simulink model "filtros_sb_r2015b"  (R2015b)
settings: Solver=VariableStepAuto  SolverMode=SingleTasking  StartTime=0.0  StopTime=10.0  RelTol=1e-3
(part 1 of 3)
settings Model: Creator=vini  LastModifiedBy=vini
settings DataIOCC: LimitDataPoints=off
settings DebuggingCC: AllowSymbolicDim=on  SFUnexpectedBacktrackingDiag=error  SFNoUnconditionalDefaultTransitionDiag=error
settings ModelReferenceCC: PropagateSignalLabelsOutOfModel=on
settings SFSimCC: SimUseLocalCustomCode=on
settings RTWCC: RTWUseLocalCustomCode=on
settings GRTTargetCC: TargetLangStandard=C99 (ISO)
settings ConfigComp: CovMetricSettings=dwe  CovHtmlReporting=off  CovSaveCumulativeToWorkspaceVar=off  CovSaveSingleToWorkspaceVar=off  CovModelRefEnable=Off  CovExternalEMLEnable=on

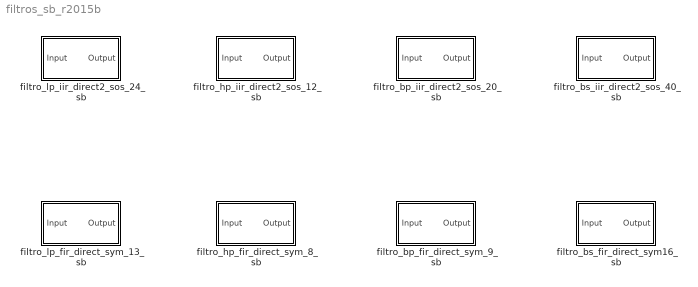
== system filtros_sb_r2015b ==
  filtro_bp_fir_direct_sym_9_sb : Subsystem  Tag=FilterWizardSubSystem
      settings: ErrorFcn=dspFilterRealizedInBasicElemsAlgLoopErrFcnCallback
  filtro_bp_iir_direct2_sos_20_sb : Subsystem  Tag=FilterWizardSubSystem
      settings: ErrorFcn=dspFilterRealizedInBasicElemsAlgLoopErrFcnCallback
  filtro_bs_fir_direct_sym16_sb : Subsystem  Tag=FilterWizardSubSystem
      settings: ErrorFcn=dspFilterRealizedInBasicElemsAlgLoopErrFcnCallback
  filtro_bs_iir_direct2_sos_40_sb : Subsystem  Tag=FilterWizardSubSystem
      settings: ErrorFcn=dspFilterRealizedInBasicElemsAlgLoopErrFcnCallback
  filtro_hp_fir_direct_sym_8_sb : Subsystem  Tag=FilterWizardSubSystem
      settings: ErrorFcn=dspFilterRealizedInBasicElemsAlgLoopErrFcnCallback
  filtro_hp_iir_direct2_sos_12_sb : Subsystem  Tag=FilterWizardSubSystem
      settings: ErrorFcn=dspFilterRealizedInBasicElemsAlgLoopErrFcnCallback
  filtro_lp_fir_direct_sym_13_sb : Subsystem  Tag=FilterWizardSubSystem
      settings: ErrorFcn=dspFilterRealizedInBasicElemsAlgLoopErrFcnCallback
  filtro_lp_iir_direct2_sos_24_sb : Subsystem  Tag=FilterWizardSubSystem
      settings: ErrorFcn=dspFilterRealizedInBasicElemsAlgLoopErrFcnCallback

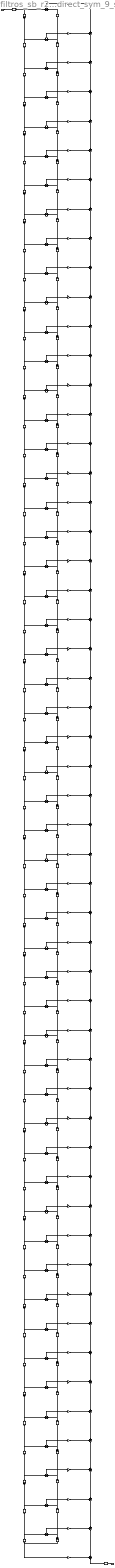
== system filtros_sb_r2015b/filtro_bp_fir_direct_sym_9_sb ==
  Input : Inport
  BodyDelayL{2..53} (52 alike) : Delay  DelayLength=1  InitialCondition=0
  BodyDelayR{2..53} (52 alike) : Delay  DelayLength=1  InitialCondition=0
  BodySumL{2..53} (52 alike) : Sum  Inputs=+|+  AccumDataTypeStr=fixdt(1,17,15)  OutDataTypeStr=fixdt(1,17,15)  RndMeth=Convergent
  BodySumR{2..53} (52 alike) : Sum  Inputs=++|  AccumDataTypeStr=fixdt(1,28,28)  OutDataTypeStr=fixdt(1,28,28)  RndMeth=Convergent
  ConvertIn : DataTypeConversion  OutDataTypeStr=fixdt(1,16,15)  RndMeth=Nearest  SaturateOnIntegerOverflow=on
  ConvertOut : DataTypeConversion  OutDataTypeStr=fixdt(1,28,28)  RndMeth=Convergent
  FootDelayL54 : Delay  DelayLength=1  InitialCondition=0
  FootSumR54 : Sum  Inputs=++|  AccumDataTypeStr=fixdt(1,28,28)  OutDataTypeStr=fixdt(1,28,28)  RndMeth=Convergent
  HeadDelayR1 : Delay  DelayLength=1  InitialCondition=0
  HeadSumL1 : Sum  Inputs=+|+  AccumDataTypeStr=fixdt(1,17,15)  OutDataTypeStr=fixdt(1,17,15)  RndMeth=Convergent
  h(1) : Gain  Gain=0.00100515299929475744  ParamDataTypeStr=fixdt(1,9,13)  OutDataTypeStr=fixdt(1,25,28)  RndMeth=Convergent
  h(10) : Gain  Gain=0.00286815818250266922  ParamDataTypeStr=fixdt(1,9,13)  OutDataTypeStr=fixdt(1,25,28)  RndMeth=Convergent
  h(11) : Gain  Gain=-0.00275820945661910556  ParamDataTypeStr=fixdt(1,9,13)  OutDataTypeStr=fixdt(1,25,28)  RndMeth=Convergent
  h(12) : Gain  Gain=-0.000348548076347779238  ParamDataTypeStr=fixdt(1,9,13)  OutDataTypeStr=fixdt(1,25,28)  RndMeth=Convergent
  h(13) : Gain  Gain=0.00308223640377106858  ParamDataTypeStr=fixdt(1,9,13)  OutDataTypeStr=fixdt(1,25,28)  RndMeth=Convergent
  h(14) : Gain  Gain=-0.00247713159189788274  ParamDataTypeStr=fixdt(1,9,13)  OutDataTypeStr=fixdt(1,25,28)  RndMeth=Convergent
  h(15) : Gain  Gain=-0.000700500797948935394  ParamDataTypeStr=fixdt(1,9,13)  OutDataTypeStr=fixdt(1,25,28)  RndMeth=Convergent
  h(16) : Gain  Gain=0.00291102947938030529  ParamDataTypeStr=fixdt(1,9,13)  OutDataTypeStr=fixdt(1,25,28)  RndMeth=Convergent
  h(17) : Gain  Gain=-0.00190512093037833075  ParamDataTypeStr=fixdt(1,9,13)  OutDataTypeStr=fixdt(1,25,28)  RndMeth=Convergent
  h(18) : Gain  Gain=-0.000876223286937654927  ParamDataTypeStr=fixdt(1,9,13)  OutDataTypeStr=fixdt(1,25,28)  RndMeth=Convergent
  h(19) : Gain  Gain=0.00226433455335455815  ParamDataTypeStr=fixdt(1,9,13)  OutDataTypeStr=fixdt(1,25,28)  RndMeth=Convergent
  h(2) : Gain  Gain=-0.00558254997081729723  ParamDataTypeStr=fixdt(1,9,13)  OutDataTypeStr=fixdt(1,25,28)  RndMeth=Convergent
  h(20) : Gain  Gain=-0.00111255989139955741  ParamDataTypeStr=fixdt(1,9,13)  OutDataTypeStr=fixdt(1,25,28)  RndMeth=Convergent
  h(21) : Gain  Gain=-0.000728999124363284351  ParamDataTypeStr=fixdt(1,9,13)  OutDataTypeStr=fixdt(1,25,28)  RndMeth=Convergent
  h(22) : Gain  Gain=0.00110819121290996431  ParamDataTypeStr=fixdt(1,9,13)  OutDataTypeStr=fixdt(1,25,28)  RndMeth=Convergent
  h(23) : Gain  Gain=-0.000227511078529173545  ParamDataTypeStr=fixdt(1,9,13)  OutDataTypeStr=fixdt(1,25,28)  RndMeth=Convergent
  h(24) : Gain  Gain=-0.000130659589522396947  ParamDataTypeStr=fixdt(1,9,13)  OutDataTypeStr=fixdt(1,25,28)  RndMeth=Convergent
  h(25) : Gain  Gain=-0.000523156580736449479  ParamDataTypeStr=fixdt(1,9,13)  OutDataTypeStr=fixdt(1,25,28)  RndMeth=Convergent
  h(26) : Gain  Gain=0.000595097230863097788  ParamDataTypeStr=fixdt(1,9,13)  OutDataTypeStr=fixdt(1,25,28)  RndMeth=Convergent
  h(27) : Gain  Gain=0.000998204699623622856  ParamDataTypeStr=fixdt(1,9,13)  OutDataTypeStr=fixdt(1,25,28)  RndMeth=Convergent
  h(28) : Gain  Gain=-0.00252037579099768623  ParamDataTypeStr=fixdt(1,9,13)  OutDataTypeStr=fixdt(1,25,28)  RndMeth=Convergent
  h(29) : Gain  Gain=0.00118419786753528396  ParamDataTypeStr=fixdt(1,9,13)  OutDataTypeStr=fixdt(1,25,28)  RndMeth=Convergent
  h(3) : Gain  Gain=-0.000115189176738601603  ParamDataTypeStr=fixdt(1,9,13)  OutDataTypeStr=fixdt(1,25,28)  RndMeth=Convergent
  h(30) : Gain  Gain=0.00267636778181485832  ParamDataTypeStr=fixdt(1,9,13)  OutDataTypeStr=fixdt(1,25,28)  RndMeth=Convergent
  h(31) : Gain  Gain=-0.00472207215493734064  ParamDataTypeStr=fixdt(1,9,13)  OutDataTypeStr=fixdt(1,25,28)  RndMeth=Convergent
  h(32) : Gain  Gain=0.0013923772800106325  ParamDataTypeStr=fixdt(1,9,13)  OutDataTypeStr=fixdt(1,25,28)  RndMeth=Convergent
  h(33) : Gain  Gain=0.00485014717213684207  ParamDataTypeStr=fixdt(1,9,13)  OutDataTypeStr=fixdt(1,25,28)  RndMeth=Convergent
  h(34) : Gain  Gain=-0.0069235701399356555  ParamDataTypeStr=fixdt(1,9,13)  OutDataTypeStr=fixdt(1,25,28)  RndMeth=Convergent
  h(35) : Gain  Gain=0.00111058492648639755  ParamDataTypeStr=fixdt(1,9,13)  OutDataTypeStr=fixdt(1,25,28)  RndMeth=Convergent
  h(36) : Gain  Gain=0.00739537400156014147  ParamDataTypeStr=fixdt(1,9,13)  OutDataTypeStr=fixdt(1,25,28)  RndMeth=Convergent
  h(37) : Gain  Gain=-0.0089146697340637248  ParamDataTypeStr=fixdt(1,9,13)  OutDataTypeStr=fixdt(1,25,28)  RndMeth=Convergent
  h(38) : Gain  Gain=0.000291547634539236929  ParamDataTypeStr=fixdt(1,9,13)  OutDataTypeStr=fixdt(1,25,28)  RndMeth=Convergent
  h(39) : Gain  Gain=0.0101165373593516666  ParamDataTypeStr=fixdt(1,9,13)  OutDataTypeStr=fixdt(1,25,28)  RndMeth=Convergent
  h(4) : Gain  Gain=0.00166912945599871393  ParamDataTypeStr=fixdt(1,9,13)  OutDataTypeStr=fixdt(1,25,28)  RndMeth=Convergent
  h(40) : Gain  Gain=-0.0104857988001575194  ParamDataTypeStr=fixdt(1,9,13)  OutDataTypeStr=fixdt(1,25,28)  RndMeth=Convergent
  h(41) : Gain  Gain=-0.00104127650841544521  ParamDataTypeStr=fixdt(1,9,13)  OutDataTypeStr=fixdt(1,25,28)  RndMeth=Convergent
  h(42) : Gain  Gain=0.0127989855562083161  ParamDataTypeStr=fixdt(1,9,13)  OutDataTypeStr=fixdt(1,25,28)  RndMeth=Convergent
  h(43) : Gain  Gain=-0.0114759563587348446  ParamDataTypeStr=fixdt(1,9,13)  OutDataTypeStr=fixdt(1,25,28)  RndMeth=Convergent
  h(44) : Gain  Gain=-0.00278510221499259731  ParamDataTypeStr=fixdt(1,9,13)  OutDataTypeStr=fixdt(1,25,28)  RndMeth=Convergent
  h(45) : Gain  Gain=0.0152021800163741443  ParamDataTypeStr=fixdt(1,9,13)  OutDataTypeStr=fixdt(1,25,28)  RndMeth=Convergent
  h(46) : Gain  Gain=-0.0117944650547391772  ParamDataTypeStr=fixdt(1,9,13)  OutDataTypeStr=fixdt(1,25,28)  RndMeth=Convergent
  h(47) : Gain  Gain=-0.0047960103156442415  ParamDataTypeStr=fixdt(1,9,13)  OutDataTypeStr=fixdt(1,25,28)  RndMeth=Convergent
  h(48) : Gain  Gain=0.0171010225526483199  ParamDataTypeStr=fixdt(1,9,13)  OutDataTypeStr=fixdt(1,25,28)  RndMeth=Convergent
  h(49) : Gain  Gain=-0.011405080653360546  ParamDataTypeStr=fixdt(1,9,13)  OutDataTypeStr=fixdt(1,25,28)  RndMeth=Convergent
  h(5) : Gain  Gain=-0.00245594406802915636  ParamDataTypeStr=fixdt(1,9,13)  OutDataTypeStr=fixdt(1,25,28)  RndMeth=Convergent
  h(50) : Gain  Gain=-0.0068708962846339202  ParamDataTypeStr=fixdt(1,9,13)  OutDataTypeStr=fixdt(1,25,28)  RndMeth=Convergent
  h(51) : Gain  Gain=0.0183207654282308771  ParamDataTypeStr=fixdt(1,9,13)  OutDataTypeStr=fixdt(1,25,28)  RndMeth=Convergent
  h(52) : Gain  Gain=-0.0103680972660661636  ParamDataTypeStr=fixdt(1,9,13)  OutDataTypeStr=fixdt(1,25,28)  RndMeth=Convergent
  h(53) : Gain  Gain=-0.00879719931139648879  ParamDataTypeStr=fixdt(1,9,13)  OutDataTypeStr=fixdt(1,25,28)  RndMeth=Convergent
  h(54) : Gain  Gain=0.0187398159211636384  ParamDataTypeStr=fixdt(1,9,13)  OutDataTypeStr=fixdt(1,25,28)  RndMeth=Convergent
  h(6) : Gain  Gain=0.000356865544766645523  ParamDataTypeStr=fixdt(1,9,13)  OutDataTypeStr=fixdt(1,25,28)  RndMeth=Convergent
  h(7) : Gain  Gain=0.00239165624029355917  ParamDataTypeStr=fixdt(1,9,13)  OutDataTypeStr=fixdt(1,25,28)  RndMeth=Convergent
  h(8) : Gain  Gain=-0.00273121981286996232  ParamDataTypeStr=fixdt(1,9,13)  OutDataTypeStr=fixdt(1,25,28)  RndMeth=Convergent
  h(9) : Gain  Gain=4.08985834428046829e-05  ParamDataTypeStr=fixdt(1,9,13)  OutDataTypeStr=fixdt(1,25,28)  RndMeth=Convergent
  Output : Outport
  wires:
  Input/1 -> ConvertIn/1
  HeadSumL1/1 -> h(1)/1
  h(1)/1 -> BodySumR2/2
  HeadDelayR1/1 -> HeadSumL1/2
  ConvertIn/1 -> HeadSumL1/1, BodyDelayL2/1
  BodyDelayL2/1 -> BodySumL2/1, BodyDelayL3/1
  BodySumL2/1 -> h(2)/1
  h(2)/1 -> BodySumR2/1
  BodyDelayR2/1 -> BodySumL2/2, HeadDelayR1/1
  BodySumR2/1 -> BodySumR3/2
  BodyDelayL3/1 -> BodySumL3/1, BodyDelayL4/1
  BodySumL3/1 -> h(3)/1
  h(3)/1 -> BodySumR3/1
  BodyDelayR3/1 -> BodySumL3/2, BodyDelayR2/1
  BodySumR3/1 -> BodySumR4/2
  BodyDelayL4/1 -> BodySumL4/1, BodyDelayL5/1
  BodySumL4/1 -> h(4)/1
  h(4)/1 -> BodySumR4/1
  BodyDelayR4/1 -> BodySumL4/2, BodyDelayR3/1
  BodySumR4/1 -> BodySumR5/2
  BodyDelayL5/1 -> BodySumL5/1, BodyDelayL6/1
  BodySumL5/1 -> h(5)/1
  h(5)/1 -> BodySumR5/1
  BodyDelayR5/1 -> BodySumL5/2, BodyDelayR4/1
  BodySumR5/1 -> BodySumR6/2
  BodyDelayL6/1 -> BodySumL6/1, BodyDelayL7/1
  BodySumL6/1 -> h(6)/1
  h(6)/1 -> BodySumR6/1
  BodyDelayR6/1 -> BodySumL6/2, BodyDelayR5/1
  BodySumR6/1 -> BodySumR7/2
  BodyDelayL7/1 -> BodySumL7/1, BodyDelayL8/1
  BodySumL7/1 -> h(7)/1
  h(7)/1 -> BodySumR7/1
  BodyDelayR7/1 -> BodySumL7/2, BodyDelayR6/1
  BodySumR7/1 -> BodySumR8/2
  BodyDelayL8/1 -> BodySumL8/1, BodyDelayL9/1
  BodySumL8/1 -> h(8)/1
  h(8)/1 -> BodySumR8/1
  BodyDelayR8/1 -> BodySumL8/2, BodyDelayR7/1
  BodySumR8/1 -> BodySumR9/2
  BodyDelayL9/1 -> BodySumL9/1, BodyDelayL10/1
  BodySumL9/1 -> h(9)/1
  h(9)/1 -> BodySumR9/1
  BodyDelayR9/1 -> BodySumL9/2, BodyDelayR8/1
  BodySumR9/1 -> BodySumR10/2
  BodyDelayL10/1 -> BodySumL10/1, BodyDelayL11/1
  BodySumL10/1 -> h(10)/1
  h(10)/1 -> BodySumR10/1
  BodyDelayR10/1 -> BodySumL10/2, BodyDelayR9/1
  BodySumR10/1 -> BodySumR11/2
  BodyDelayL11/1 -> BodySumL11/1, BodyDelayL12/1
  BodySumL11/1 -> h(11)/1
  h(11)/1 -> BodySumR11/1
  BodyDelayR11/1 -> BodySumL11/2, BodyDelayR10/1
  BodySumR11/1 -> BodySumR12/2
  BodyDelayL12/1 -> BodySumL12/1, BodyDelayL13/1
  BodySumL12/1 -> h(12)/1
  h(12)/1 -> BodySumR12/1
  BodyDelayR12/1 -> BodySumL12/2, BodyDelayR11/1
  BodySumR12/1 -> BodySumR13/2
  BodyDelayL13/1 -> BodySumL13/1, BodyDelayL14/1
  BodySumL13/1 -> h(13)/1
  h(13)/1 -> BodySumR13/1
  BodyDelayR13/1 -> BodySumL13/2, BodyDelayR12/1
  BodySumR13/1 -> BodySumR14/2
  BodyDelayL14/1 -> BodySumL14/1, BodyDelayL15/1
  BodySumL14/1 -> h(14)/1
  h(14)/1 -> BodySumR14/1
  BodyDelayR14/1 -> BodySumL14/2, BodyDelayR13/1
  BodySumR14/1 -> BodySumR15/2
  BodyDelayL15/1 -> BodySumL15/1, BodyDelayL16/1
  BodySumL15/1 -> h(15)/1
  h(15)/1 -> BodySumR15/1
  BodyDelayR15/1 -> BodySumL15/2, BodyDelayR14/1
  BodySumR15/1 -> BodySumR16/2
  BodyDelayL16/1 -> BodySumL16/1, BodyDelayL17/1
  BodySumL16/1 -> h(16)/1
  h(16)/1 -> BodySumR16/1
  BodyDelayR16/1 -> BodySumL16/2, BodyDelayR15/1
  BodySumR16/1 -> BodySumR17/2
  BodyDelayL17/1 -> BodySumL17/1, BodyDelayL18/1
  BodySumL17/1 -> h(17)/1
  h(17)/1 -> BodySumR17/1
  BodyDelayR17/1 -> BodySumL17/2, BodyDelayR16/1
  BodySumR17/1 -> BodySumR18/2
  BodyDelayL18/1 -> BodySumL18/1, BodyDelayL19/1
  BodySumL18/1 -> h(18)/1
  h(18)/1 -> BodySumR18/1
  BodyDelayR18/1 -> BodySumL18/2, BodyDelayR17/1
  BodySumR18/1 -> BodySumR19/2
  BodyDelayL19/1 -> BodySumL19/1, BodyDelayL20/1
  BodySumL19/1 -> h(19)/1
  h(19)/1 -> BodySumR19/1
  BodyDelayR19/1 -> BodySumL19/2, BodyDelayR18/1
  BodySumR19/1 -> BodySumR20/2
  BodyDelayL20/1 -> BodySumL20/1, BodyDelayL21/1
  BodySumL20/1 -> h(20)/1
  h(20)/1 -> BodySumR20/1
  BodyDelayR20/1 -> BodySumL20/2, BodyDelayR19/1
  BodySumR20/1 -> BodySumR21/2
  BodyDelayL21/1 -> BodySumL21/1, BodyDelayL22/1
  BodySumL21/1 -> h(21)/1
  h(21)/1 -> BodySumR21/1
  BodyDelayR21/1 -> BodySumL21/2, BodyDelayR20/1
  BodySumR21/1 -> BodySumR22/2
  BodyDelayL22/1 -> BodySumL22/1, BodyDelayL23/1
  BodySumL22/1 -> h(22)/1
  h(22)/1 -> BodySumR22/1
  BodyDelayR22/1 -> BodySumL22/2, BodyDelayR21/1
  BodySumR22/1 -> BodySumR23/2
  BodyDelayL23/1 -> BodySumL23/1, BodyDelayL24/1
  BodySumL23/1 -> h(23)/1
  h(23)/1 -> BodySumR23/1
  BodyDelayR23/1 -> BodySumL23/2, BodyDelayR22/1
  BodySumR23/1 -> BodySumR24/2
  BodyDelayL24/1 -> BodySumL24/1, BodyDelayL25/1
  BodySumL24/1 -> h(24)/1
  h(24)/1 -> BodySumR24/1
  BodyDelayR24/1 -> BodySumL24/2, BodyDelayR23/1
  BodySumR24/1 -> BodySumR25/2
  BodyDelayL25/1 -> BodySumL25/1, BodyDelayL26/1
  BodySumL25/1 -> h(25)/1
  h(25)/1 -> BodySumR25/1
  BodyDelayR25/1 -> BodySumL25/2, BodyDelayR24/1
  BodySumR25/1 -> BodySumR26/2
  BodyDelayL26/1 -> BodySumL26/1, BodyDelayL27/1
  BodySumL26/1 -> h(26)/1
  h(26)/1 -> BodySumR26/1
  BodyDelayR26/1 -> BodySumL26/2, BodyDelayR25/1
  BodySumR26/1 -> BodySumR27/2
  BodyDelayL27/1 -> BodySumL27/1, BodyDelayL28/1
  BodySumL27/1 -> h(27)/1
  h(27)/1 -> BodySumR27/1
  BodyDelayR27/1 -> BodySumL27/2, BodyDelayR26/1
  BodySumR27/1 -> BodySumR28/2
  BodyDelayL28/1 -> BodySumL28/1, BodyDelayL29/1
  BodySumL28/1 -> h(28)/1
  h(28)/1 -> BodySumR28/1
  BodyDelayR28/1 -> BodySumL28/2, BodyDelayR27/1
  BodySumR28/1 -> BodySumR29/2
  BodyDelayL29/1 -> BodySumL29/1, BodyDelayL30/1
  BodySumL29/1 -> h(29)/1
  h(29)/1 -> BodySumR29/1
  BodyDelayR29/1 -> BodySumL29/2, BodyDelayR28/1
  BodySumR29/1 -> BodySumR30/2
  BodyDelayL30/1 -> BodySumL30/1, BodyDelayL31/1
  BodySumL30/1 -> h(30)/1
  h(30)/1 -> BodySumR30/1
  BodyDelayR30/1 -> BodySumL30/2, BodyDelayR29/1
  BodySumR30/1 -> BodySumR31/2
  BodyDelayL31/1 -> BodySumL31/1, BodyDelayL32/1
  BodySumL31/1 -> h(31)/1
  h(31)/1 -> BodySumR31/1
  BodyDelayR31/1 -> BodySumL31/2, BodyDelayR30/1
  BodySumR31/1 -> BodySumR32/2
  BodyDelayL32/1 -> BodySumL32/1, BodyDelayL33/1
  BodySumL32/1 -> h(32)/1
  h(32)/1 -> BodySumR32/1
  BodyDelayR32/1 -> BodySumL32/2, BodyDelayR31/1
  BodySumR32/1 -> BodySumR33/2
  BodyDelayL33/1 -> BodySumL33/1, BodyDelayL34/1
  BodySumL33/1 -> h(33)/1
  h(33)/1 -> BodySumR33/1
  BodyDelayR33/1 -> BodySumL33/2, BodyDelayR32/1
  BodySumR33/1 -> BodySumR34/2
  BodyDelayL34/1 -> BodySumL34/1, BodyDelayL35/1
  BodySumL34/1 -> h(34)/1
  h(34)/1 -> BodySumR34/1
  BodyDelayR34/1 -> BodySumL34/2, BodyDelayR33/1
  BodySumR34/1 -> BodySumR35/2
  BodyDelayL35/1 -> BodySumL35/1, BodyDelayL36/1
  BodySumL35/1 -> h(35)/1
  h(35)/1 -> BodySumR35/1
  BodyDelayR35/1 -> BodySumL35/2, BodyDelayR34/1
  BodySumR35/1 -> BodySumR36/2
  BodyDelayL36/1 -> BodySumL36/1, BodyDelayL37/1
  BodySumL36/1 -> h(36)/1
  h(36)/1 -> BodySumR36/1
  BodyDelayR36/1 -> BodySumL36/2, BodyDelayR35/1
  BodySumR36/1 -> BodySumR37/2
  BodyDelayL37/1 -> BodySumL37/1, BodyDelayL38/1
  BodySumL37/1 -> h(37)/1
  h(37)/1 -> BodySumR37/1
  BodyDelayR37/1 -> BodySumL37/2, BodyDelayR36/1
  BodySumR37/1 -> BodySumR38/2
  BodyDelayL38/1 -> BodySumL38/1, BodyDelayL39/1
  BodySumL38/1 -> h(38)/1
  h(38)/1 -> BodySumR38/1
  BodyDelayR38/1 -> BodySumL38/2, BodyDelayR37/1
  BodySumR38/1 -> BodySumR39/2
  BodyDelayL39/1 -> BodySumL39/1, BodyDelayL40/1
  BodySumL39/1 -> h(39)/1
  h(39)/1 -> BodySumR39/1
  BodyDelayR39/1 -> BodySumL39/2, BodyDelayR38/1
  BodySumR39/1 -> BodySumR40/2
  BodyDelayL40/1 -> BodySumL40/1, BodyDelayL41/1
  BodySumL40/1 -> h(40)/1
  h(40)/1 -> BodySumR40/1
  BodyDelayR40/1 -> BodySumL40/2, BodyDelayR39/1
  BodySumR40/1 -> BodySumR41/2
  BodyDelayL41/1 -> BodySumL41/1, BodyDelayL42/1
  BodySumL41/1 -> h(41)/1
  h(41)/1 -> BodySumR41/1
  BodyDelayR41/1 -> BodySumL41/2, BodyDelayR40/1
  BodySumR41/1 -> BodySumR42/2
  BodyDelayL42/1 -> BodySumL42/1, BodyDelayL43/1
  BodySumL42/1 -> h(42)/1
  h(42)/1 -> BodySumR42/1
  BodyDelayR42/1 -> BodySumL42/2, BodyDelayR41/1
  BodySumR42/1 -> BodySumR43/2
  BodyDelayL43/1 -> BodySumL43/1, BodyDelayL44/1
  BodySumL43/1 -> h(43)/1
  h(43)/1 -> BodySumR43/1
  BodyDelayR43/1 -> BodySumL43/2, BodyDelayR42/1
  BodySumR43/1 -> BodySumR44/2
  BodyDelayL44/1 -> BodySumL44/1, BodyDelayL45/1
  BodySumL44/1 -> h(44)/1
  h(44)/1 -> BodySumR44/1
  BodyDelayR44/1 -> BodySumL44/2, BodyDelayR43/1
  BodySumR44/1 -> BodySumR45/2
  BodyDelayL45/1 -> BodySumL45/1, BodyDelayL46/1
  BodySumL45/1 -> h(45)/1
  h(45)/1 -> BodySumR45/1
  BodyDelayR45/1 -> BodySumL45/2, BodyDelayR44/1
  BodySumR45/1 -> BodySumR46/2
  BodyDelayL46/1 -> BodySumL46/1, BodyDelayL47/1
  BodySumL46/1 -> h(46)/1
  h(46)/1 -> BodySumR46/1
  BodyDelayR46/1 -> BodySumL46/2, BodyDelayR45/1
  BodySumR46/1 -> BodySumR47/2
  BodyDelayL47/1 -> BodySumL47/1, BodyDelayL48/1
  BodySumL47/1 -> h(47)/1
  h(47)/1 -> BodySumR47/1
  BodyDelayR47/1 -> BodySumL47/2, BodyDelayR46/1
  BodySumR47/1 -> BodySumR48/2
  BodyDelayL48/1 -> BodySumL48/1, BodyDelayL49/1
  BodySumL48/1 -> h(48)/1
  h(48)/1 -> BodySumR48/1
  BodyDelayR48/1 -> BodySumL48/2, BodyDelayR47/1
  BodySumR48/1 -> BodySumR49/2
  BodyDelayL49/1 -> BodySumL49/1, BodyDelayL50/1
  BodySumL49/1 -> h(49)/1
  h(49)/1 -> BodySumR49/1
  BodyDelayR49/1 -> BodySumL49/2, BodyDelayR48/1
  BodySumR49/1 -> BodySumR50/2
  BodyDelayL50/1 -> BodySumL50/1, BodyDelayL51/1
  BodySumL50/1 -> h(50)/1
  h(50)/1 -> BodySumR50/1
  BodyDelayR50/1 -> BodySumL50/2, BodyDelayR49/1
  BodySumR50/1 -> BodySumR51/2
  BodyDelayL51/1 -> BodySumL51/1, BodyDelayL52/1
  BodySumL51/1 -> h(51)/1
  h(51)/1 -> BodySumR51/1
  BodyDelayR51/1 -> BodySumL51/2, BodyDelayR50/1
  BodySumR51/1 -> BodySumR52/2
  BodyDelayL52/1 -> BodySumL52/1, BodyDelayL53/1
  BodySumL52/1 -> h(52)/1
  h(52)/1 -> BodySumR52/1
  BodyDelayR52/1 -> BodySumL52/2, BodyDelayR51/1
  BodySumR52/1 -> BodySumR53/2
  BodyDelayL53/1 -> BodySumL53/1, FootDelayL54/1
  BodySumL53/1 -> h(53)/1
  h(53)/1 -> BodySumR53/1
  BodyDelayR53/1 -> BodySumL53/2, BodyDelayR52/1
  BodySumR53/1 -> FootSumR54/2
  FootDelayL54/1 -> h(54)/1, BodyDelayR53/1
  h(54)/1 -> FootSumR54/1
  FootSumR54/1 -> ConvertOut/1
  ConvertOut/1 -> Output/1

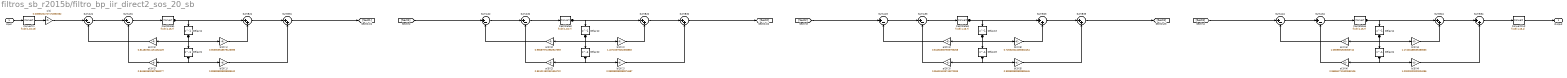
== system filtros_sb_r2015b/filtro_bp_iir_direct2_sos_20_sb ==
  Input : Inport
  CastState{1..4} (4 alike) : DataTypeConversion  OutDataTypeStr=fixdt(1,16,7)  RndMeth=Convergent
  ConvertIn : DataTypeConversion  OutDataTypeStr=fixdt(1,16,15)  RndMeth=Nearest  SaturateOnIntegerOverflow=on
  ConvertOut : DataTypeConversion  OutDataTypeStr=fixdt(1,16,4)  RndMeth=Convergent
  Delay{11..14,21..24} (8 alike) : Delay  DelayLength=1  InitialCondition=0
  SumA{21..24,31..34} (8 alike) : Sum  Inputs=|+-  AccumDataTypeStr=fixdt(1,40,26)  OutDataTypeStr=fixdt(1,40,26)  RndMeth=Convergent
  SumB{21..24,31..34} (8 alike) : Sum  Inputs=|++  AccumDataTypeStr=fixdt(1,40,26)  OutDataTypeStr=fixdt(1,40,26)  RndMeth=Convergent
  a(2)(1) : Gain  Gain=0.814819011151262429  ParamDataTypeStr=fixdt(0,20,19)  OutDataTypeStr=fixdt(1,36,26)  RndMeth=Convergent
  a(2)(2) : Gain  Gain=0.965879710982947559  ParamDataTypeStr=fixdt(0,20,19)  OutDataTypeStr=fixdt(1,36,26)  RndMeth=Convergent
  a(2)(3) : Gain  Gain=0.812603367593793258  ParamDataTypeStr=fixdt(0,20,19)  OutDataTypeStr=fixdt(1,36,26)  RndMeth=Convergent
  a(2)(4) : Gain  Gain=1.0659691505063742  ParamDataTypeStr=fixdt(0,20,19)  OutDataTypeStr=fixdt(1,36,26)  RndMeth=Convergent
  a(3)(1) : Gain  Gain=0.843633602697968277  ParamDataTypeStr=fixdt(0,20,19)  OutDataTypeStr=fixdt(1,36,26)  RndMeth=Convergent
  a(3)(2) : Gain  Gain=0.851011920331394722  ParamDataTypeStr=fixdt(0,20,19)  OutDataTypeStr=fixdt(1,36,26)  RndMeth=Convergent
  a(3)(3) : Gain  Gain=0.954924333743372933  ParamDataTypeStr=fixdt(0,20,19)  OutDataTypeStr=fixdt(1,36,26)  RndMeth=Convergent
  a(3)(4) : Gain  Gain=0.958842711800593106  ParamDataTypeStr=fixdt(0,20,19)  OutDataTypeStr=fixdt(1,36,26)  RndMeth=Convergent
  b(2)(1) : Gain  Gain=0.353353948679126395  ParamDataTypeStr=fixdt(0,20,19)  OutDataTypeStr=fixdt(1,36,26)  RndMeth=Convergent
  b(2)(2) : Gain  Gain=1.40715579232338883  ParamDataTypeStr=fixdt(0,20,19)  OutDataTypeStr=fixdt(1,36,26)  RndMeth=Convergent
  b(2)(3) : Gain  Gain=0.725520024065602454  ParamDataTypeStr=fixdt(0,20,19)  OutDataTypeStr=fixdt(1,36,26)  RndMeth=Convergent
  b(2)(4) : Gain  Gain=1.17400488535383563  ParamDataTypeStr=fixdt(0,20,19)  OutDataTypeStr=fixdt(1,36,26)  RndMeth=Convergent
  b(3)(1) : Gain  Gain=0.999999999999989342  ParamDataTypeStr=fixdt(0,20,19)  OutDataTypeStr=fixdt(1,36,26)  RndMeth=Convergent
  b(3)(2) : Gain  Gain=0.999999999999974687  ParamDataTypeStr=fixdt(0,20,19)  OutDataTypeStr=fixdt(1,36,26)  RndMeth=Convergent
  b(3)(3) : Gain  Gain=0.999999999999999445  ParamDataTypeStr=fixdt(0,20,19)  OutDataTypeStr=fixdt(1,36,26)  RndMeth=Convergent
  b(3)(4) : Gain  Gain=1.00000000000004086  ParamDataTypeStr=fixdt(0,20,19)  OutDataTypeStr=fixdt(1,36,26)  RndMeth=Convergent
  s(1) : Gain  Gain=0.00853204727172851562  ParamDataTypeStr=fixdt(0,20,26)  OutDataTypeStr=fixdt(1,16,10)  RndMeth=Convergent
  Output : Outport
  wires:
  Input/1 -> ConvertIn/1
  s(1)/1 -> SumA21/1
  SumA21/1 -> SumA31/1
  SumA31/1 -> CastState1/1
  CastState1/1 -> SumB21/1, Delay11/1
  SumB21/1 -> SumB31/1
  SumB31/1 -> [Sect1]
  a(2)(1)/1 -> SumA21/2
  Delay11/1 -> a(2)(1)/1, b(2)(1)/1, Delay21/1
  b(2)(1)/1 -> SumB21/2
  a(3)(1)/1 -> SumA31/2
  Delay21/1 -> a(3)(1)/1, b(3)(1)/1
  b(3)(1)/1 -> SumB31/2
  ConvertIn/1 -> s(1)/1
  [Sect1] -> SumA22/1
  SumA22/1 -> SumA32/1
  SumA32/1 -> CastState2/1
  CastState2/1 -> SumB22/1, Delay12/1
  SumB22/1 -> SumB32/1
  SumB32/1 -> [Sect2]
  a(2)(2)/1 -> SumA22/2
  Delay12/1 -> a(2)(2)/1, b(2)(2)/1, Delay22/1
  b(2)(2)/1 -> SumB22/2
  a(3)(2)/1 -> SumA32/2
  Delay22/1 -> a(3)(2)/1, b(3)(2)/1
  b(3)(2)/1 -> SumB32/2
  [Sect2] -> SumA23/1
  SumA23/1 -> SumA33/1
  SumA33/1 -> CastState3/1
  CastState3/1 -> SumB23/1, Delay13/1
  SumB23/1 -> SumB33/1
  SumB33/1 -> [Sect3]
  a(2)(3)/1 -> SumA23/2
  Delay13/1 -> a(2)(3)/1, b(2)(3)/1, Delay23/1
  b(2)(3)/1 -> SumB23/2
  a(3)(3)/1 -> SumA33/2
  Delay23/1 -> a(3)(3)/1, b(3)(3)/1
  b(3)(3)/1 -> SumB33/2
  [Sect3] -> SumA24/1
  SumA24/1 -> SumA34/1
  SumA34/1 -> CastState4/1
  CastState4/1 -> SumB24/1, Delay14/1
  SumB24/1 -> SumB34/1
  SumB34/1 -> ConvertOut/1
  a(2)(4)/1 -> SumA24/2
  Delay14/1 -> a(2)(4)/1, b(2)(4)/1, Delay24/1
  b(2)(4)/1 -> SumB24/2
  a(3)(4)/1 -> SumA34/2
  Delay24/1 -> a(3)(4)/1, b(3)(4)/1
  b(3)(4)/1 -> SumB34/2
  ConvertOut/1 -> Output/1
